simulink model "Dynamic_Calculations"  (R2018a)
settings: Solver=ode3  StartTime=0.0  StopTime=0.06  RelTol=1e-3  EnableMultiTasking=on
libraries: hdlsllib x4, simulink x1
settings Model: Creator=Estra  LastModifiedBy=Talha Rao
settings SolverCC: PositivePriorityOrder=on
settings DataIOCC: LimitDataPoints=on  SaveFormat=Array  SaveOutput=off  SaveTime=off
settings OptimizationCC: BlockReduction=off  ConditionallyExecuteInputs=off  DefaultParameterBehavior=Inlined  UseDivisionForNetSlopeComputation=on  UseFloatMulNetSlope=on  InlineInvariantSignals=on  PassReuseOutputArgsAs=Individual arguments  ExpressionDepthLimit=2147483647  ZeroExternalMemoryAtStartup=off  ZeroInternalMemoryAtStartup=off  NoFixptDivByZeroProtection=on  EfficientFloat2IntCast=on  LifeSpan=1  MaxStackSize=64
settings DebuggingCC: SignalInfNanChecking=warning  UnderspecifiedInitializationDetection=Classic  MergeDetectMultiDrivingBlocksExec=none  SolverPrmCheckMsg=warning  ParameterTunabilityLossMsg=error  UniqueDataStoreMsg=warning  AllowSymbolicDim=off  StateNameClashWarn=warning  SFUnexpectedBacktrackingDiag=warning  SFNoUnconditionalDefaultTransitionDiag=warning  SFExecutionAtInitializationDiag=none
settings HardwareCC: ProdBitPerPointer=32  ProdBitPerSizeT=32  ProdBitPerPtrDiffT=32  ProdLargestAtomicInteger=Long  ProdLargestAtomicFloat=Double  ProdWordSize=32  ProdLongLongMode=on  ProdHWDeviceType=ARM Compatible->ARM Cortex  TargetBitPerPointer=64  TargetBitPerSizeT=64  TargetBitPerPtrDiffT=64  TargetLongLongMode=on  TargetIntDivRoundTo=Zero  TargetEndianess=LittleEndian  TargetWordSize=64  TargetHWDeviceType=Custom Processor->MATLAB Host Computer  ProdEqTarget=off
settings ModelReferenceCC: PropagateSignalLabelsOutOfModel=off
settings SFSimCC: MATLABDynamicMemAlloc=off
settings RTWCC: SystemTargetFile=ert.tlc  HardwareBoard=Xilinx Zynq-7000 based board  TLCOptions="-aInlineSetEventsForThisBaseRateFcn=TLC_FALSE -aSuppressMultiTaskScheduler=TLC_FALSE  -aRateBasedStepFcn=0"  TemplateMakefile=ert_default_tmf  GenerateReport=on  Toolchain=Xilinx Software Development Kit (SDK)  IncludeHyperlinkInReport=on  LaunchReport=on  GenerateTraceInfo=on  GenerateTraceReport=on  GenerateTraceReportSl=on  GenerateTraceReportSf=on  GenerateTraceReportEml=on  GenerateCodeMetricsReport=on
settings CodeAppCC: ForceParamTrailComments=on  IgnoreCustomStorageClasses=off  OperatorAnnotations=on  SimulinkDataObjDesc=on  SFDataObjDesc=on  CustomSymbolStrGlobalVar=rt$N$M  CustomSymbolStrType=$N$M  CustomSymbolStrFcn=$N$M$F  CustomSymbolStrMacro=$N$M  InsertBlockDesc=on
settings ERTTargetCC: IncludeMdlTerminateFcn=off  CombineSignalStateStructs=on  SupportAbsoluteTime=off  SupportComplex=off  SupportNonInlinedSFcns=on  SupportVariableSizeSignals=on  InlinedParameterPlacement=NonHierarchical  ERTFilePackagingFormat=CompactWithDataFile
settings ConfigComp: CovMetricSettings=dw  CovHtmlReporting=on  CovSaveCumulativeToWorkspaceVar=on  CovSaveSingleToWorkspaceVar=on  CovExternalEMLEnable=off

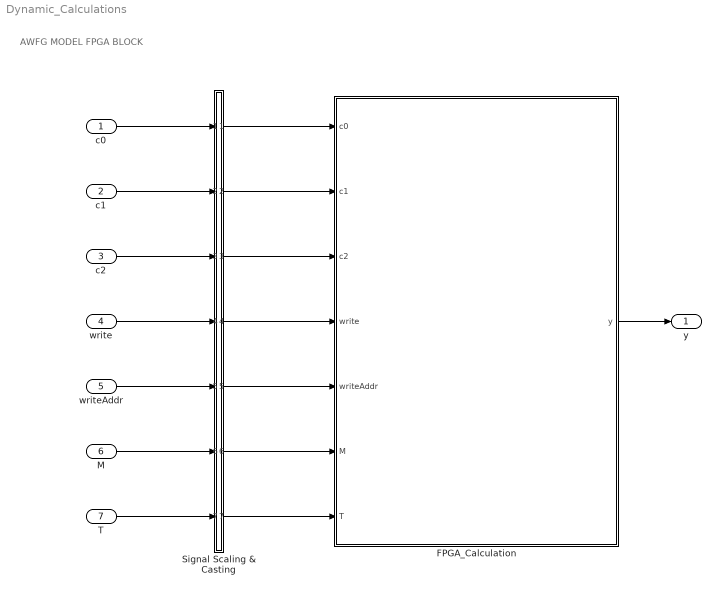
== system Dynamic_Calculations ==
  note: AWFG MODEL FPGA BLOCK
  c0 : Inport  OutDataTypeStr=int32  PortDimensions=[1 1]  SampleTime=[1e-08,0]
  c1 : Inport  Port=2  OutDataTypeStr=int32  PortDimensions=[1 1]  SampleTime=[1e-08,0]
  c2 : Inport  Port=3  OutDataTypeStr=int32  PortDimensions=[1 1]  SampleTime=[1e-08,0]
  write : Inport  Port=4  OutDataTypeStr=boolean  PortDimensions=[1 1]  SampleTime=[1e-08,0]
  writeAddr : Inport  Port=5  OutDataTypeStr=uint8  PortDimensions=[1 1]  SampleTime=[1e-08,0]
  M : Inport  Port=6  OutDataTypeStr=int32  PortDimensions=1  SampleTime=[1e-08,0]
  T : Inport  Port=7  OutDataTypeStr=uint32  PortDimensions=1
  FPGA_Calculation : Subsystem
  Signal Scaling & Casting : Subsystem
  y : Outport  OutDataTypeStr=fixdt(1,27,19)  PortDimensions=[1 1]  SampleTime=[1e-08,0]
  wires:
  FPGA_Calculation/1(y) -> y/1
  c0/1 -> Signal Scaling & Casting/1(c0)
  c1/1 -> Signal Scaling & Casting/2(c1)
  c2/1 -> Signal Scaling & Casting/3(c2)
  write/1 -> Signal Scaling & Casting/4(write)
  writeAddr/1 -> Signal Scaling & Casting/5(writeAddr)
  T/1 -> Signal Scaling & Casting/7(T)
  Signal Scaling & Casting/6(Mi) -> FPGA_Calculation/6(M)
  Signal Scaling & Casting/7(Ti) -> FPGA_Calculation/7(T)
  Signal Scaling & Casting/5(writeAddri) -> FPGA_Calculation/5(writeAddr)
  Signal Scaling & Casting/4(writei) -> FPGA_Calculation/4(write)
  Signal Scaling & Casting/3(c2i) -> FPGA_Calculation/3(c2)
  Signal Scaling & Casting/2(c1i) -> FPGA_Calculation/2(c1)
  Signal Scaling & Casting/1(c0i) -> FPGA_Calculation/1(c0)
  M/1 -> Signal Scaling & Casting/6(M)

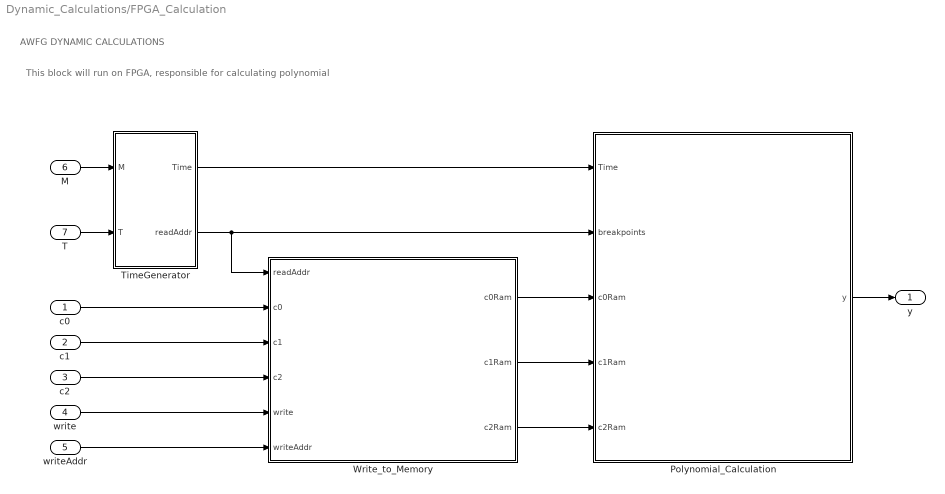
== system Dynamic_Calculations/FPGA_Calculation ==
  note: This block will run on FPGA, responsible for calculating polynomial
  note: AWFG DYNAMIC CALCULATIONS
  c0 : Inport
  c1 : Inport  Port=2
  c2 : Inport  Port=3
  write : Inport  Port=4
  writeAddr : Inport  Port=5
  M : Inport  Port=6
  T : Inport  Port=7
  Polynomial_Calculation : Subsystem
  TimeGenerator : Subsystem
  Write_to_Memory : Subsystem
  y : Outport
  wires:
  TimeGenerator/1(Time) -> Polynomial_Calculation/1(Time)
  Write_to_Memory/2(c1Ram) -> Polynomial_Calculation/4(c1Ram)
  writeAddr/1 -> Write_to_Memory/6(writeAddr)
  write/1 -> Write_to_Memory/5(write)
  Write_to_Memory/3(c2Ram) -> Polynomial_Calculation/5(c2Ram)
  M/1 -> TimeGenerator/1(M)
  TimeGenerator/2(readAddr) -> Polynomial_Calculation/2(breakpoints), Write_to_Memory/1(readAddr)
  Write_to_Memory/1(c0Ram) -> Polynomial_Calculation/3(c0Ram)
  T/1 -> TimeGenerator/2(T)
  c2/1 -> Write_to_Memory/4(c2)
  Polynomial_Calculation/1(y) -> y/1
  c0/1 -> Write_to_Memory/2(c0)
  c1/1 -> Write_to_Memory/3(c1)

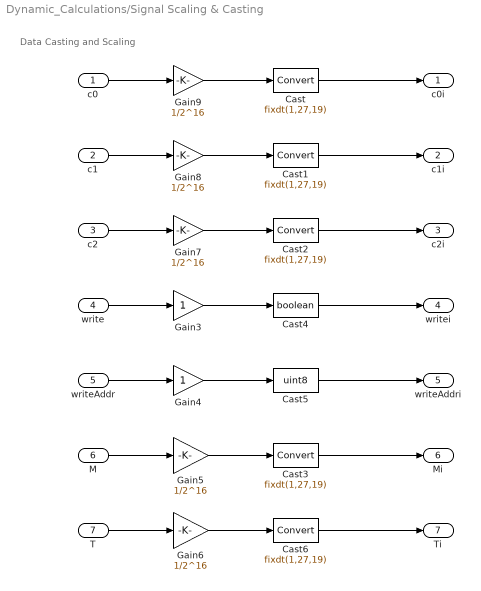
== system Dynamic_Calculations/Signal Scaling & Casting ==
  note: Data Casting and Scaling
  c0 : Inport
  c1 : Inport  Port=2
  c2 : Inport  Port=3
  write : Inport  Port=4
  writeAddr : Inport  Port=5
  M : Inport  Port=6
  T : Inport  Port=7
  Cast{,1..3,6} (5 alike) : DataTypeConversion  OutDataTypeStr=fixdt(1,27,19)
  Cast4 : DataTypeConversion  OutDataTypeStr=boolean
  Cast5 : DataTypeConversion  OutDataTypeStr=uint8
  Gain3 : Gain
  Gain4 : Gain
  Gain{5..9} (5 alike) : Gain  Gain=1/2^16
  c0i : Outport
  c1i : Outport  Port=2
  c2i : Outport  Port=3
  writei : Outport  Port=4
  writeAddri : Outport  Port=5
  Mi : Outport  Port=6
  Ti : Outport  Port=7
  wires:
  Cast3/1 -> Mi/1
  Cast/1 -> c0i/1
  Cast1/1 -> c1i/1
  Cast2/1 -> c2i/1
  Cast4/1 -> writei/1
  Cast5/1 -> writeAddri/1
  Cast6/1 -> Ti/1
  Gain6/1 -> Cast6/1
  Gain5/1 -> Cast3/1
  Gain4/1 -> Cast5/1
  Gain3/1 -> Cast4/1
  Gain7/1 -> Cast2/1
  Gain8/1 -> Cast1/1
  Gain9/1 -> Cast/1
  T/1 -> Gain6/1
  M/1 -> Gain5/1
  writeAddr/1 -> Gain4/1
  write/1 -> Gain3/1
  c2/1 -> Gain7/1
  c1/1 -> Gain8/1
  c0/1 -> Gain9/1

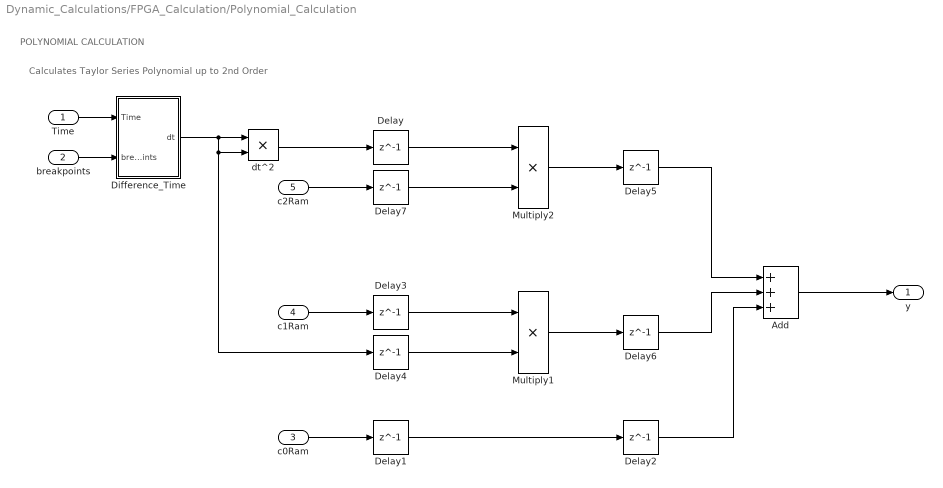
== system Dynamic_Calculations/FPGA_Calculation/Polynomial_Calculation ==
  note: Calculates Taylor Series Polynomial up to 2nd Order
  note: POLYNOMIAL CALCULATION
  Time : Inport
  breakpoints : Inport  Port=2
  c0Ram : Inport  Port=3
  c1Ram : Inport  Port=4
  c2Ram : Inport  Port=5
  Add : Sum  Inputs=3  OutDataTypeStr=fixdt(1,27,19)
  Delay{,1..7} (8 alike) : Delay  DelayLength=1
  Difference_Time : Subsystem
  Multiply1 : Product  OutDataTypeStr=fixdt(1,27,19)
  Multiply2 : Product  OutDataTypeStr=fixdt(1,27,19)  InputSameDT=on
  dt^2 : Product  OutDataTypeStr=fixdt(1,27,19)
  y : Outport
  wires:
  Add/1 -> y/1
  breakpoints/1 -> Difference_Time/2(breakpoints)
  Time/1 -> Difference_Time/1(Time)
  Difference_Time/1(dt) -> Delay4/1, dt^2/2, dt^2/1
  Delay2/1 -> Add/3
  Delay6/1 -> Add/2
  Delay5/1 -> Add/1
  Delay7/1 -> Multiply2/2
  Multiply2/1 -> Delay5/1
  Multiply1/1 -> Delay6/1
  Delay/1 -> Multiply2/1
  c2Ram/1 -> Delay7/1
  Delay4/1 -> Multiply1/2
  Delay3/1 -> Multiply1/1
  c1Ram/1 -> Delay3/1
  Delay1/1 -> Delay2/1
  c0Ram/1 -> Delay1/1
  dt^2/1 -> Delay/1

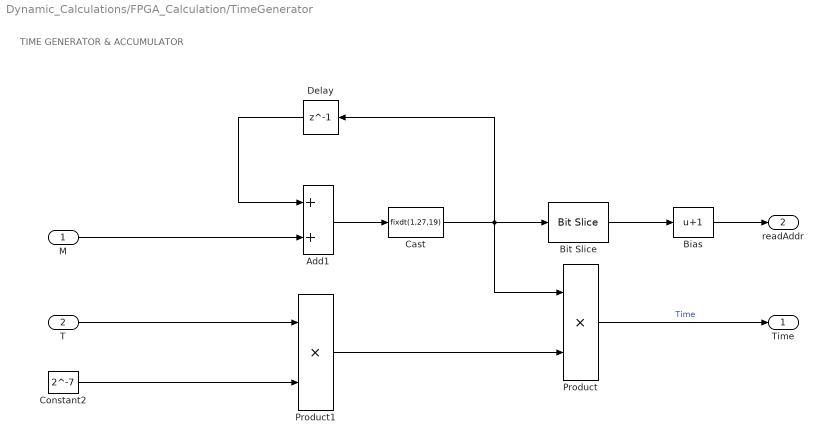
== system Dynamic_Calculations/FPGA_Calculation/TimeGenerator ==
  note: TIME GENERATOR & ACCUMULATOR
  M : Inport
  T : Inport  Port=2
  Add1 : Sum  OutDataTypeStr=fixdt(0,26,19)
  Bias : Bias  Bias=1
  Bit Slice : hdlsllib/Logic and Bit Operations/Bit Slice  lidx=26  ridx=19
  Cast : DataTypeConversion  OutDataTypeStr=fixdt(1,27,19)
  Constant2 : Constant  Value=2^-7  OutDataTypeStr=fixdt(1,27,19)
  Delay : Delay  DelayLength=1
  Product : Product  OutDataTypeStr=fixdt(1,27,19)
  Product1 : Product  OutDataTypeStr=fixdt(1,27,19)
  Time : Outport
  readAddr : Outport  Port=2
  wires:
  Constant2/1 -> Product1/2
  Bias/1 -> readAddr/1
  Cast/1 -> Delay/1, Product/1, Bit Slice/1
  Delay/1 -> Add1/1
  T/1 -> Product1/1
  M/1 -> Add1/2
  Bit Slice/1 -> Bias/1
  Add1/1 -> Cast/1
  Product1/1 -> Product/2
  Product/1 -> Time/1  "Time"

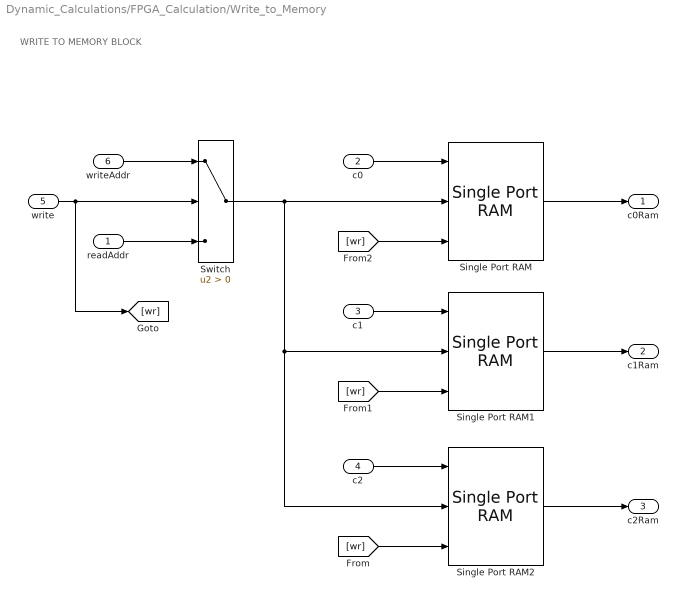
== system Dynamic_Calculations/FPGA_Calculation/Write_to_Memory ==
  note: WRITE TO MEMORY BLOCK
  readAddr : Inport
  c0 : Inport  Port=2
  c1 : Inport  Port=3
  c2 : Inport  Port=4
  write : Inport  Port=5
  writeAddr : Inport  Port=6
  Single Port RAM : hdlsllib/HDL RAMs/Single Port RAM  ram_size=8  dout_type=New data
      settings: SourceProductName=HDL Coder  SourceProductBaseCode=HD
  Single Port RAM1 : hdlsllib/HDL RAMs/Single Port RAM  ram_size=8  dout_type=New data
      settings: SourceProductName=HDL Coder  SourceProductBaseCode=HD
  Single Port RAM2 : hdlsllib/HDL RAMs/Single Port RAM  ram_size=8  dout_type=New data
      settings: SourceProductName=HDL Coder  SourceProductBaseCode=HD
  Switch : Switch  Criteria=u2 > Threshold
  c0Ram : Outport
  c1Ram : Outport  Port=2
  c2Ram : Outport  Port=3
  wires:
  c2/1 -> Single Port RAM2/1
  c1/1 -> Single Port RAM1/1
  c0/1 -> Single Port RAM/1
  Single Port RAM2/1 -> c2Ram/1
  Single Port RAM1/1 -> c1Ram/1
  [wr] -> Single Port RAM2/3
  [wr] -> Single Port RAM1/3
  readAddr/1 -> Switch/3
  writeAddr/1 -> Switch/1
  write/1 -> Switch/2, [wr]
  [wr] -> Single Port RAM/3
  Switch/1 -> Single Port RAM1/2, Single Port RAM2/2, Single Port RAM/2
  Single Port RAM/1 -> c0Ram/1

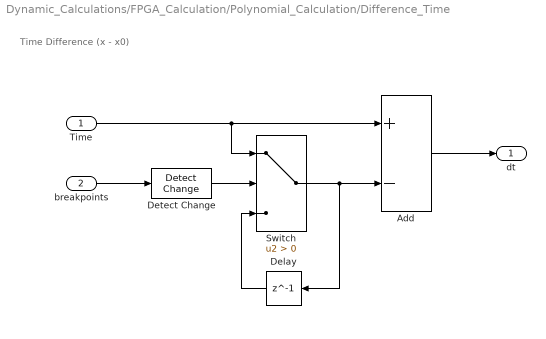
== system Dynamic_Calculations/FPGA_Calculation/Polynomial_Calculation/Difference_Time ==
  note: Time Difference (x - x0)
  Time : Inport
  breakpoints : Inport  Port=2
  Add : Sum  Inputs=+-  OutDataTypeStr=fixdt(1,27,19)
  Delay : Delay  DelayLength=1
  Detect Change : simulink/Logic and Bit Operations/Detect Change  vinit=0  OutDataTypeStr=boolean
  Switch : Switch  Criteria=u2 > Threshold
  dt : Outport
  wires:
  Add/1 -> dt/1
  Detect Change/1 -> Switch/2
  Delay/1 -> Switch/3
  breakpoints/1 -> Detect Change/1
  Time/1 -> Add/1, Switch/1
  Switch/1 -> Add/2, Delay/1
